simulink model "basic_model"  (R2023a)
settings: Solver=VariableStepAuto  StartTime=0.0  StopTime=20  RelTol=1e-3
settings Model: Creator=pc  LastModifiedBy=pc

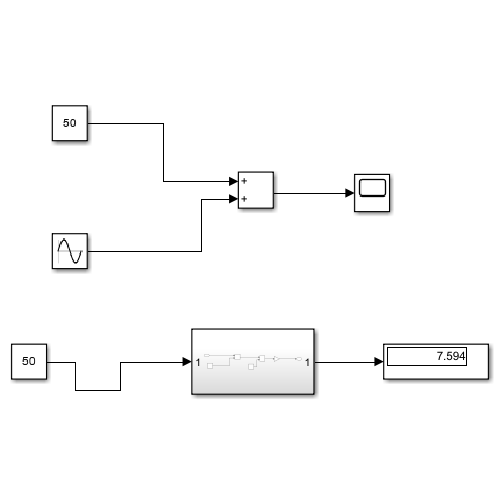
[thumbnail: Simulink's stored preview of the top-level diagram]
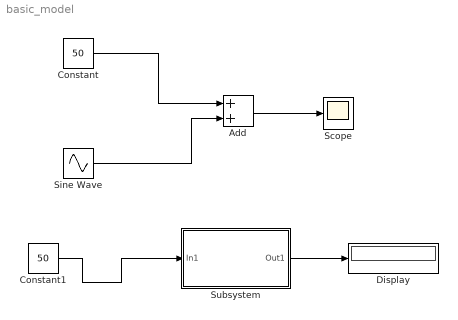
== system basic_model ==
  Add : Sum
  Constant : Constant  Value=50
  Constant1 : Constant  Value=50
  Display : Display
  Scope : Scope
  Sine Wave : Sin  Amplitude=5  Frequency=2*pi/24  SampleTime=0
  Subsystem : Subsystem
  wires:
  Constant/1 -> Add/1
  Sine Wave/1 -> Add/2
  Add/1 -> Scope/1
  Subsystem/1(Out1) -> Display/1
  Constant1/1 -> Subsystem/1(In1)

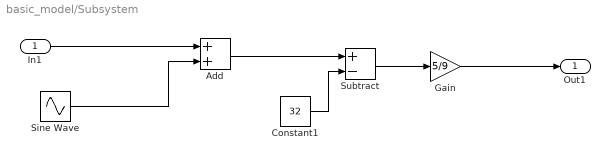
== system basic_model/Subsystem ==
  In1 : Inport
  Add : Sum
  Constant1 : Constant  Value=32
  Gain : Gain  Gain=5/9
  Sine Wave : Sin  Amplitude=5  Frequency=2*pi/24  SampleTime=0
  Subtract : Sum  Inputs=+-
  Out1 : Outport
  wires:
  Subtract/1 -> Gain/1
  Constant1/1 -> Subtract/2
  Gain/1 -> Out1/1
  Sine Wave/1 -> Add/2
  In1/1 -> Add/1
  Add/1 -> Subtract/1
